simulink model "px4demo_attitude_systemtest11"  (R2016b)
settings: Solver=FixedStepDiscrete  StartTime=0.0  StopTime=inf  RelTol=1e-3
PostLoadFcn:
  | kFactor = 1.2;
  | 
  | KpRollAttitude = 0.630138625117681 / kFactor;
  | KiRollAttitude = 0.0552303199591522 / kFactor;
  | 
  | KpPitchAttitude = 0.630138625117681 / kFactor;
  | KiPitchAttitude = 0.0552303199591522 / kFactor;
  | 
  | KpRollRate = 1.31533836563383 / kFactor;
  | KiRollRate = 0.460338699849681 / kFactor;
  | 
  | KpPitchRate = 1.31533836563383 / kFactor;
  | KiPitchRate = 0.460338699849681 / kFactor;
  | 
  | KpYawRate = 1.31533836563383 / kFactor;
  | KiYawRate = 0.460338699849681 / kFactor;
undefined symbols (not defined in the file or in its folder): PX4_TUNE_ENUM, RGBLED_COLOR_ENUM, RGBLED_MODE_ENUM
libraries: pixhawk_slib_sensors_actuators x4, simulink x1, pixhawk_slib_ADC_serial x1
settings Model: SimulationMode=external  Creator=Steve  LastModifiedBy=E6320
settings SolverCC: AutoInsertRateTranBlk=on
settings DataIOCC: LimitDataPoints=on  SaveFormat=Array
settings OptimizationCC: DefaultParameterBehavior=Inlined  LifeSpan=1  MaxStackSize=64
settings DebuggingCC: SolverPrmCheckMsg=warning  AllowSymbolicDim=off  SFUnexpectedBacktrackingDiag=warning  SFNoUnconditionalDefaultTransitionDiag=warning  SFExecutionAtInitializationDiag=none
settings HardwareCC: ProdBitPerPointer=32  ProdBitPerSizeT=32  ProdBitPerPtrDiffT=32  ProdLargestAtomicInteger=Long  ProdLargestAtomicFloat=Double  ProdWordSize=32  ProdHWDeviceType=ARM Compatible->ARM Cortex
settings ModelReferenceCC: PropagateSignalLabelsOutOfModel=off
settings RTWCC: SystemTargetFile=ert.tlc  HardwareBoard=Pixhawk PX4  TemplateMakefile=ert_default_tmf  Description=Embedded Coder  GenerateReport=on  Toolchain=Pixhawk Toolchain  IncludeHyperlinkInReport=on  LaunchReport=on  GenerateTraceReport=on  GenerateTraceReportSl=on  GenerateTraceReportSf=on  GenerateTraceReportEml=on  GenerateCodeMetricsReport=on
settings CodeAppCC: IgnoreCustomStorageClasses=off
settings ERTTargetCC: CodeReplacementLibrary=GCC ARM Cortex-A9  SupportContinuousTime=on  ExtMode=on  ExtModeTransport=1  ExtModeMexFile=ext_serial_win32_comm  ExtModeMexArgs=1 7 115200 10  ERTCustomFileTemplate=PX4_codertarget_file_process.tlc  ConvertIfToSwitch=off  SuppressUnreachableDefaultCases=off
settings ConfigComp: CovMetricSettings=dw  CovHtmlReporting=on  CovSaveCumulativeToWorkspaceVar=on  CovSaveSingleToWorkspaceVar=on  CovExternalEMLEnable=off  CovSFcnEnable=off

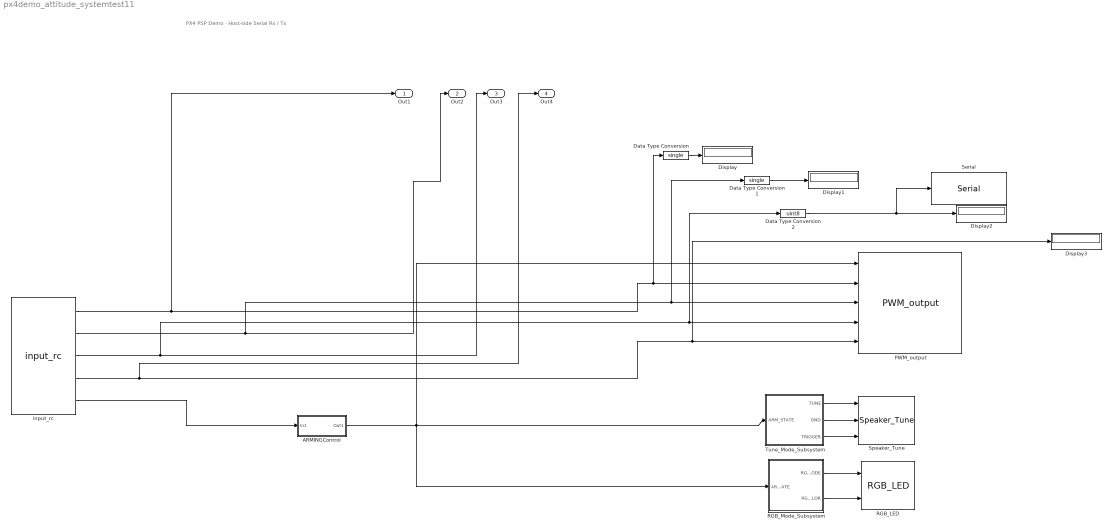
== system px4demo_attitude_systemtest11 ==
  note: PX4 PSP Demo - Host-side Serial Rx / Tx
  ARMINGControl : Subsystem
  Data Type Conversion : DataTypeConversion  OutDataTypeStr=single
  Data Type Conversion1 : DataTypeConversion  OutDataTypeStr=single
  Data Type Conversion2 : DataTypeConversion  OutDataTypeStr=uint8
  Display{,1..3} (4 alike) : Display
  PWM_output : pixhawk_slib_sensors_actuators/PWM_output  pwm_rate=400Hz  show_pwm1=on  show_pwm2=on  show_pwm3=on  show_pwm4=on  show_pwm5=off  show_pwm6=off  show_pwm7=off  show_pwm8=off
  RGB_LED : pixhawk_slib_sensors_actuators/RGB_LED
  RGB_Mode_Subsystem : Subsystem
  Serial : pixhawk_slib_ADC_serial/Serial  DeviceName=/dev/ttyACM0  ReadOrWrite=Writing  BaudRateStr=57600  block=on  WriteStatus=on  Terminator=off  Header=off  NumBytesRead=4  TerminatorChar=\n  HeaderData=[ uint8( hex2dec( 'DE' ) ), uint8( hex2dec( 'AD' ) ), uint8( hex2dec( 'C0' ) ), uint8( hex2dec( 'DE' ) ) ]  SimulateUsing=Code generation
  Speaker_Tune : pixhawk_slib_sensors_actuators/Speaker_Tune
  Tune_Mode_Subsystem : Subsystem
  input_rc : pixhawk_slib_sensors_actuators/input_rc  sampletime=1/250  channel1=on  channel2=on  channel3=on  channel4=on  channel5=on  channel6=off  channel7=off  channel8=off  ch_count=off  rssi=off  rc_failsafe=off  rc_lost=off  rc_inputsource=off
  Out1 : Outport
  Out2 : Outport  Port=2
  Out3 : Outport  Port=3
  Out4 : Outport  Port=4
  wires:
  RGB_Mode_Subsystem/1(RGB_MODE) -> RGB_LED/1
  RGB_Mode_Subsystem/2(RGB_COLOR) -> RGB_LED/2
  Tune_Mode_Subsystem/1(TUNE) -> Speaker_Tune/1
  Tune_Mode_Subsystem/2(GND) -> Speaker_Tune/2
  Tune_Mode_Subsystem/3(TRIGGER) -> Speaker_Tune/3
  ARMINGControl/1(Out1) -> PWM_output/1, Tune_Mode_Subsystem/1(ARM_STATE), RGB_Mode_Subsystem/1(ARM_STATE)
  input_rc/5 -> ARMINGControl/1(In1)
  input_rc/3 -> Out3/1, Data Type Conversion2/1, PWM_output/4
  input_rc/1 -> Out1/1, Data Type Conversion/1, PWM_output/2
  input_rc/2 -> Out2/1, Data Type Conversion1/1, PWM_output/3
  input_rc/4 -> Out4/1, Display3/1, PWM_output/5
  Data Type Conversion/1 -> Display/1
  Data Type Conversion1/1 -> Display1/1
  Data Type Conversion2/1 -> Serial/1, Display2/1

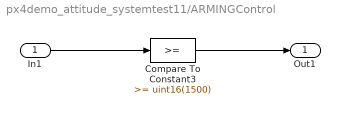
== system px4demo_attitude_systemtest11/ARMINGControl ==
  In1 : Inport
  Compare To Constant3 : simulink/Logic and Bit Operations/Compare To Constant  relop=>=  const=uint16(1500)  OutDataTypeStr=boolean
  Out1 : Outport
  wires:
  Compare To Constant3/1 -> Out1/1
  In1/1 -> Compare To Constant3/1

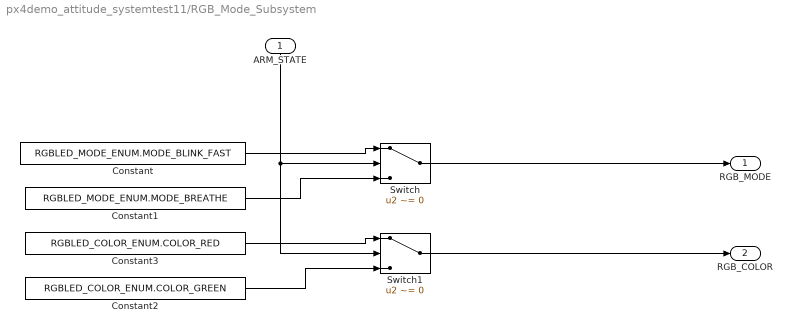
== system px4demo_attitude_systemtest11/RGB_Mode_Subsystem ==
  ARM_STATE : Inport
  Constant : Constant  Value=RGBLED_MODE_ENUM.MODE_BLINK_FAST  OutDataTypeStr=Enum: RGBLED_MODE_ENUM
  Constant1 : Constant  Value=RGBLED_MODE_ENUM.MODE_BREATHE  OutDataTypeStr=Enum: RGBLED_MODE_ENUM
  Constant2 : Constant  Value=RGBLED_COLOR_ENUM.COLOR_GREEN  OutDataTypeStr=Enum: RGBLED_COLOR_ENUM
  Constant3 : Constant  Value=RGBLED_COLOR_ENUM.COLOR_RED  OutDataTypeStr=Enum: RGBLED_COLOR_ENUM
  Switch : Switch  Criteria=u2 ~= 0  Threshold=1500  SampleTime=1/2
  Switch1 : Switch  Criteria=u2 ~= 0  Threshold=1500  SampleTime=1/2
  RGB_MODE : Outport
  RGB_COLOR : Outport  Port=2
  wires:
  ARM_STATE/1 -> Switch1/2, Switch/2
  Constant/1 -> Switch/1
  Constant1/1 -> Switch/3
  Switch/1 -> RGB_MODE/1
  Constant3/1 -> Switch1/1
  Constant2/1 -> Switch1/3
  Switch1/1 -> RGB_COLOR/1

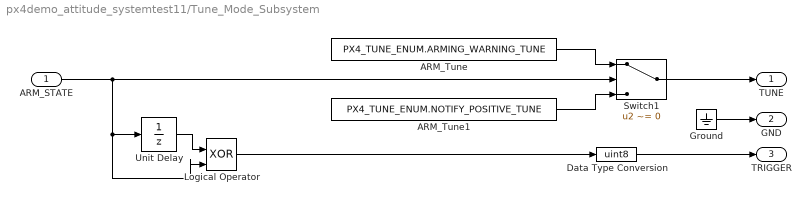
== system px4demo_attitude_systemtest11/Tune_Mode_Subsystem ==
  ARM_STATE : Inport
  ARM_Tune : Constant  Value=PX4_TUNE_ENUM.ARMING_WARNING_TUNE  OutDataTypeStr=Enum: PX4_TUNE_ENUM
  ARM_Tune1 : Constant  Value=PX4_TUNE_ENUM.NOTIFY_POSITIVE_TUNE  OutDataTypeStr=Enum: PX4_TUNE_ENUM
  Data Type Conversion : DataTypeConversion  OutDataTypeStr=uint8
  Ground : Ground
  Logical Operator : Logic  Operator=XOR  IconShape=distinctive  AllPortsSameDT=off  OutDataTypeStr=boolean
  Switch1 : Switch  Criteria=u2 ~= 0  Threshold=1500
  Unit Delay : UnitDelay  SampleTime=-1
  TUNE : Outport
  GND : Outport  Port=2
  TRIGGER : Outport  Port=3
  wires:
  Ground/1 -> GND/1
  Data Type Conversion/1 -> TRIGGER/1
  Switch1/1 -> TUNE/1
  ARM_Tune/1 -> Switch1/1
  ARM_Tune1/1 -> Switch1/3
  ARM_STATE/1 -> Logical Operator/2, Unit Delay/1, Switch1/2
  Unit Delay/1 -> Logical Operator/1
  Logical Operator/1 -> Data Type Conversion/1
